simulink model "c28x_spi_eeprom_interrupt"  (R2021b)
settings: Solver=FixedStepDiscrete  StartTime=0.0  StopTime=inf  RelTol=1e-3  EnableMultiTasking=on
libraries: c280xlib x6, simulink x5, svdutilitieslib x2, c2000lib x1, demo_controls x1
settings Model: SimulationMode=external  ExtModeTrigDuration=8  Creator=The MathWorks, Inc.  LastModifiedBy=The MathWorks, Inc.
settings SolverCC: AlgebraicLoopSolver=TrustRegion  DecoupledContinuousIntegration=on  MinimalZcImpactIntegration=on
settings DataIOCC: ReturnWorkspaceOutputs=off
settings OptimizationCC: DefaultUnderspecifiedDataType=single  EnhancedBackFolding=on  PassReuseOutputArgsAs=Individual arguments  MaxStackSize=512  OptimizeBlockOrder=speed  DifferentSizesBufferReuse=on  OptimizationCustomize=off  EfficientTunableParamExpr=on
settings DebuggingCC: InheritedTsInSrcMsg=none  MultiTaskDSMMsg=none  ParameterTunabilityLossMsg=error  SFMachineParentedDataDiag=warning  ArithmeticOperatorsInVariantConditions=warning
settings HardwareCC: ProdBitPerChar=16  ProdBitPerInt=16  ProdBitPerPointer=32  ProdBitPerSizeT=32  ProdBitPerPtrDiffT=32  ProdLargestAtomicInteger=Integer  ProdLargestAtomicFloat=None  ProdWordSize=16  ProdLongLongMode=on  ProdHWDeviceType=Texas Instruments->C2000
settings SFSimCC: SimUseLocalCustomCode=off  MATLABDynamicMemAlloc=off  CustomCodeUndefinedFunction=UseInterfaceOnly
settings RTWCC: Description=Embedded Coder  SystemTargetFile=ert.tlc  HardwareBoard=TI Delfino F28379D LaunchPad  TemplateMakefile=ert_default_tmf  GenerateReport=on  RTWUseLocalCustomCode=off  Toolchain=Texas Instruments Code Composer Studio (C2000)  IncludeHyperlinkInReport=on  LaunchReport=on  GenerateTraceInfo=on  GenerateTraceReport=on  GenerateTraceReportSl=on  GenerateTraceReportSf=on  GenerateTraceReportEml=on
settings CodeAppCC: ForceParamTrailComments=on  IgnoreCustomStorageClasses=off  OperatorAnnotations=on  SimulinkDataObjDesc=on  SFDataObjDesc=on  InsertBlockDesc=on
settings ERTTargetCC: CodeReplacementLibrary=TI C28x  ExtModeTransport=4  ExtModeStaticAlloc=on  ExtModeStaticAllocSize=10000  ExtModeMexFile=ext_xcp  ExtModeIntrfLevel=Level2 - Open

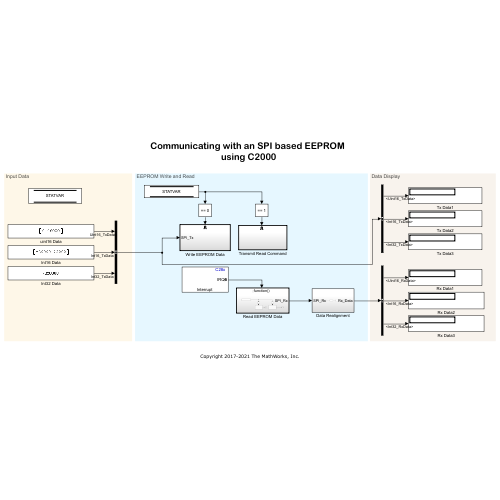
[thumbnail: Simulink's stored preview of the top-level diagram]
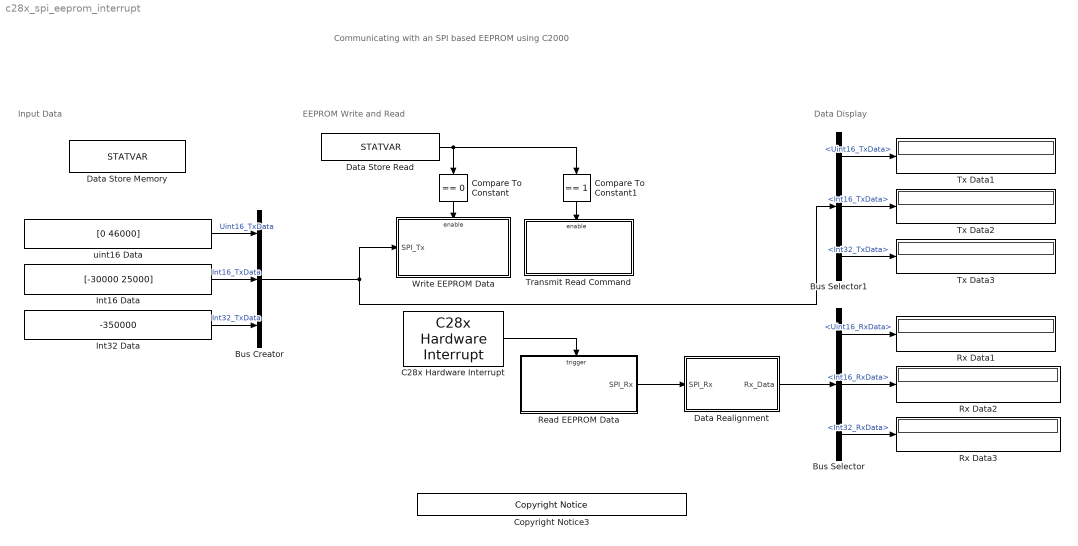
== system c28x_spi_eeprom_interrupt ==
  note: Communicating with an SPI based EEPROM
      | using C2000
  note: Input Data
  note: EEPROM Write and Read
  note: Data Display
  Bus Creator : BusCreator  Inputs=3
  Bus Selector : BusSelector  OutputSignals=Uint16_RxData,Int16_RxData,Int32_RxData
  Bus Selector1 : BusSelector  OutputSignals=Uint16_TxData,Int16_TxData,Int32_TxData
  C28x Hardware Interrupt : c2000lib/Scheduling/C28x Hardware Interrupt  irqnumbers=6  pienumbers=1  irqpriorities=30  irqpreempts=1  showinput=off  dspchiptype=C280X
      settings: SourceProductBaseCode=TIC2000
  Compare To Constant : simulink/Logic and Bit Operations/Compare To Constant  relop===  const=0  OutDataTypeStr=boolean  ZeroCross=off
  Compare To Constant1 : simulink/Logic and Bit Operations/Compare To Constant  relop===  const=1  OutDataTypeStr=boolean  ZeroCross=off
  Copyright Notice3 : demo_controls/Copyright Notice  year=2017  prod=tic2000
      settings: SourceProductBaseCode=ME
  Data Realignment : Subsystem
  Data Store Memory : DataStoreMemory  DataStoreName=STATVAR  ShowAdditionalParam=off  OutDataTypeStr=uint16
  Data Store Read : DataStoreRead  DataStoreName=STATVAR  IndexOptions=Index vector (dialog)  Indices=1  OutputSizes=1
  Int16 Data : Constant  Value=[-30000 25000]  OutDataTypeStr=int16  SampleTime=-1
  Int32 Data : Constant  Value=-350000  OutDataTypeStr=int32  SampleTime=-1
  Read EEPROM Data : Subsystem
  Rx Data1 : Display
  Rx Data2 : Display
  Rx Data3 : Display
  Transmit Read Command : Subsystem  TreatAsAtomicUnit=on
  Tx Data1 : Display
  Tx Data2 : Display
  Tx Data3 : Display
  Write EEPROM Data : Subsystem
  uint16 Data : Constant  Value=[0 46000]  OutDataTypeStr=uint16  SampleTime=-1
  wires:
  Compare To Constant/1 -> Write EEPROM Data/Enable
  Bus Selector/1 -> Rx Data1/1  "<Uint16_RxData>"
  Read EEPROM Data/1(SPI_Rx) -> Data Realignment/1(SPI_Rx)
  Bus Creator/1 -> Bus Selector1/1, Write EEPROM Data/1(SPI_Tx)
  Bus Selector1/3 -> Tx Data3/1  "<Int32_TxData>"
  Bus Selector1/1 -> Tx Data1/1  "<Uint16_TxData>"
  Int32 Data/1 -> Bus Creator/3  "Int32_TxData"
  Data Realignment/1(Rx_Data) -> Bus Selector/1
  uint16 Data/1 -> Bus Creator/1  "Uint16_TxData"
  C28x Hardware Interrupt/1 -> Read EEPROM Data/Trigger
  Data Store Read/1 -> Compare To Constant1/1, Compare To Constant/1
  Compare To Constant1/1 -> Transmit Read Command/Enable
  Bus Selector/2 -> Rx Data2/1  "<Int16_RxData>"
  Bus Selector1/2 -> Tx Data2/1  "<Int16_TxData>"
  Int16 Data/1 -> Bus Creator/2  "Int16_TxData"
  Bus Selector/3 -> Rx Data3/1  "<Int32_RxData>"

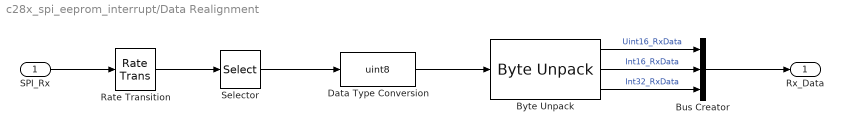
== system c28x_spi_eeprom_interrupt/Data Realignment ==
  SPI_Rx : Inport
  Bus Creator : BusCreator  Inputs=3
  Byte Unpack : svdutilitieslib/Byte Unpack  dimensions={2,2,1}  datatypes={'uint16','int16','int32'}  byteAlign=1  blockPlatform=arduinoert
      settings: SourceProductBaseCode=ANDROID,ARDUINO,ML_ARDUINO,ECCORTEXA,ECCORTEXR,SC_BEAGLEBONE_BLUE,EC_FREEDOM_BOARD,EC_FRDM_K64F,INTEL_BLOCKSET,MICROBIT,NUCLEO,NVIDIA,PX4AUTOPILOTS,RASPPIIO,STMICRODIS,TIC2000,XILINX_BLOCKSET
  Data Type Conversion : DataTypeConversion  OutDataTypeStr=uint8
  Rate Transition : RateTransition  Deterministic=off  OutPortSampleTime=0.2
  Selector : Selector  InputPortWidth=15  IndexOptions=Index vector (dialog)  Indices=[4:15]  OutputSizes=1
  Rx_Data : Outport  InitialOutput=0  VectorParamsAs1DForOutWhenUnconnected=off
  wires:
  Selector/1 -> Data Type Conversion/1
  Data Type Conversion/1 -> Byte Unpack/1
  Byte Unpack/2 -> Bus Creator/2  "Int16_RxData"
  Byte Unpack/3 -> Bus Creator/3  "Int32_RxData"
  Rate Transition/1 -> Selector/1
  Bus Creator/1 -> Rx_Data/1
  SPI_Rx/1 -> Rate Transition/1
  Byte Unpack/1 -> Bus Creator/1  "Uint16_RxData"

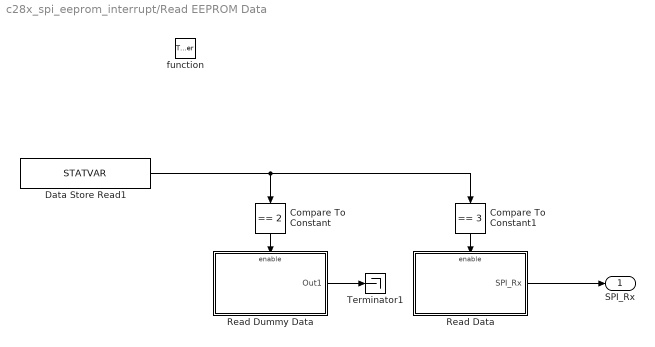
== system c28x_spi_eeprom_interrupt/Read EEPROM Data ==
  function : TriggerPort  TriggerType=function-call  VariantControl=Variant
  Compare To Constant : simulink/Logic and Bit Operations/Compare To Constant  relop===  const=2  OutDataTypeStr=boolean  ZeroCross=off
  Compare To Constant1 : simulink/Logic and Bit Operations/Compare To Constant  relop===  const=3  OutDataTypeStr=boolean  ZeroCross=off
  Data Store Read1 : DataStoreRead  DataStoreName=STATVAR  IndexOptions=Index vector (dialog)  Indices=1  OutputSizes=1
  Read Data : Subsystem
  Read Dummy Data : Subsystem
  Terminator1 : Terminator
  SPI_Rx : Outport  VectorParamsAs1DForOutWhenUnconnected=off
  wires:
  Data Store Read1/1 -> Compare To Constant/1, Compare To Constant1/1
  Read Data/1(SPI_Rx) -> SPI_Rx/1
  Compare To Constant1/1 -> Read Data/Enable
  Compare To Constant/1 -> Read Dummy Data/Enable
  Read Dummy Data/1(Out1) -> Terminator1/1

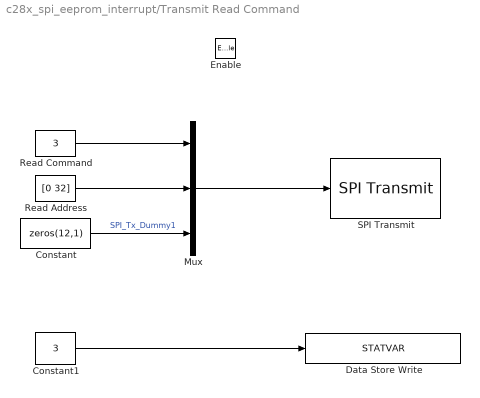
== system c28x_spi_eeprom_interrupt/Transmit Read Command ==
  Enable : EnablePort
  Constant : Constant  Value=zeros(12,1)  OutDataTypeStr=uint16  SampleTime=-1
  Constant1 : Constant  Value=3  OutDataTypeStr=uint16  SampleTime=-1
  Data Store Write : DataStoreWrite  DataStoreName=STATVAR  IndexOptions=Index vector (dialog)  Indices=1  OutputSizes=1
  Mux : Mux  Inputs=3
  Read Address : Constant  Value=[0 32]  OutDataTypeStr=uint16  SampleTime=-1
  Read Command : Constant  Value=3  OutDataTypeStr=uint16  SampleTime=-1
  SPI Transmit : c280xlib/SPI Transmit  Priority=1  SPISelect=SPI_A  ClockPolarity=Rising_edge  ClockPhase=Delay_half_cycle  SPIModule=uint32(0)  Mode=Master  BusSpeed=uint32(1000000)  FirstBitToTransfer=Most significant bit (MSB)  ClockMode=0  BlockFunction=Write  EnableRegisterAddress=on  RegisterAddress=0  OutputDataType=int8  OutputDataLength=1  BlockingMode=on  DataBits=8  UseCustomSSPin=Explicit GPIO calls  ActiveLowSSPin=Active low  Pin=1
      settings: SourceProductBaseCode=TIC2000
  wires:
  Read Address/1 -> Mux/2
  Constant/1 -> Mux/3  "SPI_Tx_Dummy1"
  Mux/1 -> SPI Transmit/1
  Read Command/1 -> Mux/1
  Constant1/1 -> Data Store Write/1

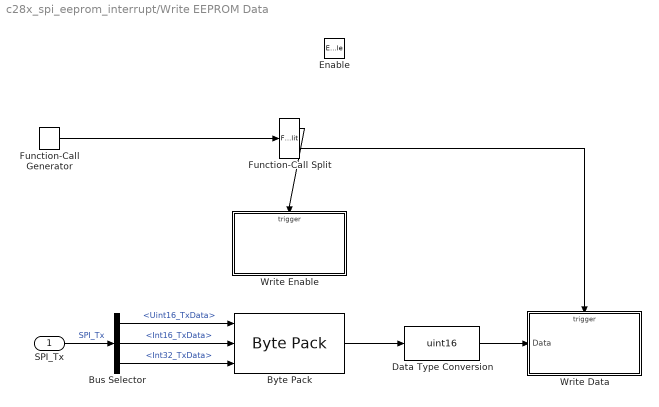
== system c28x_spi_eeprom_interrupt/Write EEPROM Data ==
  SPI_Tx : Inport
  Enable : EnablePort
  Bus Selector : BusSelector  OutputSignals=Uint16_TxData,Int16_TxData,Int32_TxData
  Byte Pack : svdutilitieslib/Byte Pack  maskPackedDataType=uint8  datatypes={'uint16','int16','int32'}  byteAlign=1  blockPlatform=arduinoert
      settings: SourceProductBaseCode=ANDROID,ARDUINO,ML_ARDUINO,ECCORTEXA,ECCORTEXR,SC_BEAGLEBONE_BLUE,EC_FREEDOM_BOARD,EC_FRDM_K64F,INTEL_BLOCKSET,MICROBIT,NUCLEO,NVIDIA,PX4AUTOPILOTS,RASPPIIO,STMICRODIS,TIC2000,XILINX_BLOCKSET
  Data Type Conversion : DataTypeConversion  OutDataTypeStr=uint16
  Function-Call Generator : simulink/Ports & Subsystems/Function-Call Generator  sample_time=-1  numberOfIterations=1  DisallowWideOutput=off
  Function-Call Split : FunctionCallSplit  NumOutputPorts=2
  Write Data : Subsystem
  Write Enable : Subsystem
  wires:
  Function-Call Generator/1 -> Function-Call Split/1
  Function-Call Split/1 -> Write Enable/Trigger
  Function-Call Split/2 -> Write Data/Trigger
  SPI_Tx/1 -> Bus Selector/1  "SPI_Tx"
  Data Type Conversion/1 -> Write Data/1(Data)
  Byte Pack/1 -> Data Type Conversion/1
  Bus Selector/1 -> Byte Pack/1  "<Uint16_TxData>"
  Bus Selector/2 -> Byte Pack/2  "<Int16_TxData>"
  Bus Selector/3 -> Byte Pack/3  "<Int32_TxData>"

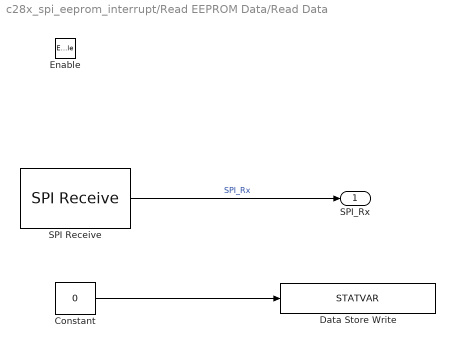
== system c28x_spi_eeprom_interrupt/Read EEPROM Data/Read Data ==
  Enable : EnablePort
  Constant : Constant  Value=0  OutDataTypeStr=uint16  SampleTime=-1
  Data Store Write : DataStoreWrite  DataStoreName=STATVAR  IndexOptions=Index vector (dialog)  Indices=1  OutputSizes=1
  SPI Receive : c280xlib/SPI Receive  Priority=2  SPISelect=SPI_A  ClockPolarity=Rising_edge  ClockPhase=Delay_half_cycle  SPIModule=uint32(0)  Mode=Master  BusSpeed=uint32(1000000)  FirstBitToTransfer=Most significant bit (MSB)  ClockMode=0  BlockFunction=Read  EnableRegisterAddress=on  RegisterAddress=0  OutputDataType=uint16  OutputDataLength=15  BlockingMode=on  SampleTime=-1  DataBits=8  UseCustomSSPin=Explicit GPIO calls  ActiveLowSSPin=Active low  Pin=1
      settings: SourceProductBaseCode=TIC2000
  SPI_Rx : Outport  VectorParamsAs1DForOutWhenUnconnected=off
  wires:
  SPI Receive/1 -> SPI_Rx/1  "SPI_Rx"
  Constant/1 -> Data Store Write/1

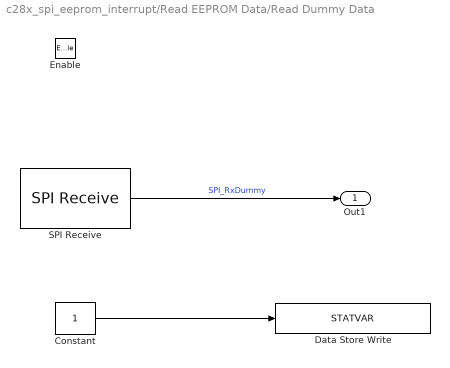
== system c28x_spi_eeprom_interrupt/Read EEPROM Data/Read Dummy Data ==
  Enable : EnablePort
  Constant : Constant  OutDataTypeStr=uint16  SampleTime=-1
  Data Store Write : DataStoreWrite  DataStoreName=STATVAR  IndexOptions=Index vector (dialog)  Indices=1  OutputSizes=1
  SPI Receive : c280xlib/SPI Receive  Priority=2  SPISelect=SPI_A  ClockPolarity=Rising_edge  ClockPhase=Delay_half_cycle  SPIModule=uint32(0)  Mode=Master  BusSpeed=uint32(1000000)  FirstBitToTransfer=Most significant bit (MSB)  ClockMode=0  BlockFunction=Read  EnableRegisterAddress=on  RegisterAddress=0  OutputDataType=uint16  OutputDataLength=15  BlockingMode=on  SampleTime=-1  DataBits=8  UseCustomSSPin=Explicit GPIO calls  ActiveLowSSPin=Active low  Pin=1
      settings: SourceProductBaseCode=TIC2000
  Out1 : Outport  VectorParamsAs1DForOutWhenUnconnected=off
  wires:
  SPI Receive/1 -> Out1/1  "SPI_RxDummy"
  Constant/1 -> Data Store Write/1

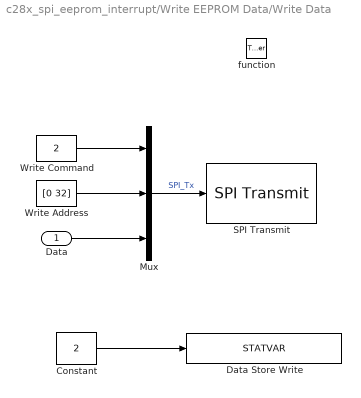
== system c28x_spi_eeprom_interrupt/Write EEPROM Data/Write Data ==
  Data : Inport
  function : TriggerPort  TriggerType=function-call  VariantControl=Variant
  Constant : Constant  Value=2  OutDataTypeStr=uint16  SampleTime=-1
  Data Store Write : DataStoreWrite  DataStoreName=STATVAR  IndexOptions=Index vector (dialog)  Indices=1  OutputSizes=1
  Mux : Mux  Inputs=3
  SPI Transmit : c280xlib/SPI Transmit  Priority=1  SPISelect=SPI_A  ClockPolarity=Rising_edge  ClockPhase=Delay_half_cycle  SPIModule=uint32(0)  Mode=Master  BusSpeed=uint32(1000000)  FirstBitToTransfer=Most significant bit (MSB)  ClockMode=0  BlockFunction=Write  EnableRegisterAddress=on  RegisterAddress=0  OutputDataType=int8  OutputDataLength=1  BlockingMode=on  DataBits=8  UseCustomSSPin=Explicit GPIO calls  ActiveLowSSPin=Active low  Pin=1
      settings: SourceProductBaseCode=TIC2000
  Write Address : Constant  Value=[0 32]  OutDataTypeStr=uint16  SampleTime=-1
  Write Command : Constant  Value=2  OutDataTypeStr=uint16  SampleTime=-1
  wires:
  Write Command/1 -> Mux/1
  Write Address/1 -> Mux/2
  Data/1 -> Mux/3
  Mux/1 -> SPI Transmit/1  "SPI_Tx"
  Constant/1 -> Data Store Write/1

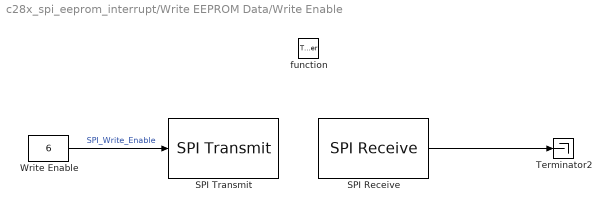
== system c28x_spi_eeprom_interrupt/Write EEPROM Data/Write Enable ==
  function : TriggerPort  TriggerType=function-call  VariantControl=Variant
  SPI Receive : c280xlib/SPI Receive  Priority=2  SPISelect=SPI_A  ClockPolarity=Rising_edge  ClockPhase=Delay_half_cycle  SPIModule=uint32(0)  Mode=Master  BusSpeed=uint32(1000000)  FirstBitToTransfer=Most significant bit (MSB)  ClockMode=0  BlockFunction=Read  EnableRegisterAddress=on  RegisterAddress=0  OutputDataType=uint16  OutputDataLength=1  BlockingMode=on  SampleTime=-1  DataBits=8  UseCustomSSPin=Explicit GPIO calls  ActiveLowSSPin=Active low  Pin=1
      settings: SourceProductBaseCode=TIC2000
  SPI Transmit : c280xlib/SPI Transmit  Priority=1  SPISelect=SPI_A  ClockPolarity=Rising_edge  ClockPhase=Delay_half_cycle  SPIModule=uint32(0)  Mode=Master  BusSpeed=uint32(1000000)  FirstBitToTransfer=Most significant bit (MSB)  ClockMode=0  BlockFunction=Write  EnableRegisterAddress=on  RegisterAddress=0  OutputDataType=int8  OutputDataLength=1  BlockingMode=on  DataBits=8  UseCustomSSPin=Explicit GPIO calls  ActiveLowSSPin=Active low  Pin=1
      settings: SourceProductBaseCode=TIC2000
  Terminator2 : Terminator
  Write Enable : Constant  Value=6  OutDataTypeStr=uint16  SampleTime=-1
  wires:
  SPI Receive/1 -> Terminator2/1
  Write Enable/1 -> SPI Transmit/1  "SPI_Write_Enable"
